simulink model "untitled"  (R2016a)
settings: Solver=VariableStepAuto  StartTime=0.0  StopTime=10.0  RelTol=1e-3
undefined symbols (not defined in the file or in its folder): k1, k2
settings Model: Creator=Marcelo  LastModifiedBy=Marcelo

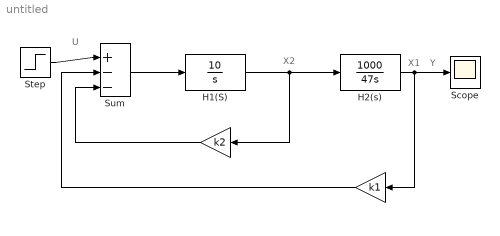
== system untitled ==
  note: U
  note: Y
  note: X1
  note: X2
  " " : Gain  Gain=k1
  " " : Gain  Gain=k2
  H1(S) : TransferFcn  Numerator=[10]  Denominator=[1 0]
  H2(s) : TransferFcn  Numerator=[1000]  Denominator=[47 0]
  Scope : Scope
  Step : Step  SampleTime=0
  Sum : Sum  Inputs=|+--
  wires:
  Step/1 -> Sum/1
  Sum/1 -> H1(S)/1
  H1(S)/1 -> " "/1, H2(s)/1
  H2(s)/1 -> Scope/1, " "/1
  " "/1 -> Sum/3
  " "/1 -> Sum/2
